simulink model "sfediticon"  (R2017b)
settings: Solver=FixedStepDiscrete  StartTime=0.0  StopTime=inf  RelTol=1e-3  EnableMultiTasking=on
CloseFcn:
  | sf_edit_icon('kill');
settings Model: FPTRunName=Active  ExtModeTrigMode=oneshot  ExtModeArmWhenConnect=off  ExtModeAutoUpdateStatusClock=off  Creator=The MathWorks, Inc.  LastModifiedBy=The MathWorks, Inc.
settings DataIOCC: SaveFormat=Array  SaveOutput=off  SaveTime=off
settings OptimizationCC: BooleanDataType=off  ExpressionDepthLimit=2147483647  InitFltsAndDblsToZero=on  EfficientMapNaN2IntZero=off  LifeSpan=inf
settings DebuggingCC: SaveWithParameterizedLinksMsg=none  UnderspecifiedInitializationDetection=Classic  MergeDetectMultiDrivingBlocksExec=none  SignalResolutionControl=TryResolveAllWithWarning  MultiTaskDSMMsg=warning  MultiTaskCondExecSysMsg=none  FcnCallInpInsideContextMsg=warning  StateNameClashWarn=warning  StrictBusMsg=None  SFUnexpectedBacktrackingDiag=warning  SFNoUnconditionalDefaultTransitionDiag=warning  SFExecutionAtInitializationDiag=none
settings HardwareCC: ProdBitPerPointer=32  ProdBitPerSizeT=32  ProdBitPerPtrDiffT=32  ProdLargestAtomicFloat=None  ProdIntDivRoundTo=Undefined  ProdEndianess=Unspecified  ProdWordSize=32  ProdHWDeviceType=32-bit Generic  TargetUnknown=on
settings ModelReferenceCC: PropagateSignalLabelsOutOfModel=off
settings SFSimCC: SimCustomHeaderCode=#define IS_MEX_TARGET 0  SimParseCustomCode=off
settings CodeAppCC: StateflowObjectComments=on
settings GRTTargetCC: TargetFcnLib=ansi_tfl_tmw.mat  TargetLangStandard=C89/C90 (ANSI)  GeneratePreprocessorConditionals=Disable all  CombineOutputUpdateFcns=off  GRTInterface=on
settings ConfigComp: CovMetricSettings=dcmtr  CovHtmlReporting=on  CovSaveCumulativeToWorkspaceVar=on  CovSaveSingleToWorkspaceVar=on  CovExternalEMLEnable=off  CovSFcnEnable=off

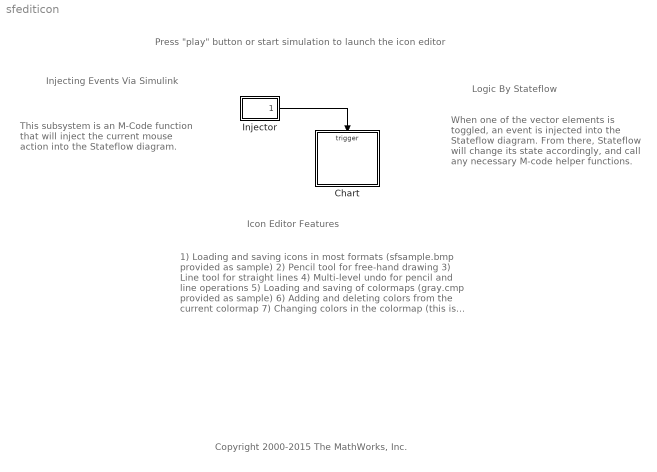
== system sfediticon ==
  note: This subsystem is an M-Code
      | function that will inject the
      | current mouse action into the
      | Stateflow diagram.
  note: Injecting Events
      | Via Simulink
  note: When one of the vector elements
      | is toggled, an event is injected
      | into the Stateflow diagram.
      | From there, Stateflow will
      | change its state accordingly,
      | and call any necessary M-code
      | helper functions.
  note: Logic By Stateflow
  note: 1) Loading and saving icons in most formats
      |      (sfsample.bmp provided as sample)
      | 2) Pencil tool for free-hand drawing
      | 3) Line tool for straight lines
      | 4) Multi-level undo for pencil and line operations
      | 5) Loading and saving of colormaps
      |      (gray.cmp provided as sample)
      | 6) Adding and deleting colors from the current
      |      colormap
      | 7) Changing colors in the colormap
      |     (this is immediately reflected in the icon)
  note: Icon Editor Features
  note: Press "play" button or start simulation to launch the icon editor
  note: Copyright 2000-2015 The MathWorks, Inc.
  Chart : Stateflow chart  TreatAsAtomicUnit=on
  Injector : Subsystem
  wires:
  Injector/1(Event) -> Chart/Trigger

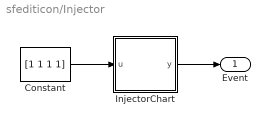
== system sfediticon/Injector ==
  Constant : Constant  Value=[1 1 1 1]
  InjectorChart : Stateflow chart  TreatAsAtomicUnit=on
  Event : Outport
  wires:
  InjectorChart/1(y) -> Event/1
  Constant/1 -> InjectorChart/1(u)

== stateflow chart sfediticon/Chart ==
  settings: executeAtInitialization=1
  state Main [parallel]
    settings: executionOrder=1
    state LineDraw
      en: ml.sf_edit_icon('anchor_line');
      du: ml.sf_edit_icon('render_line');
      ex:  ml.sf_edit_icon('commit');
    state Idle
    state PencilDraw
      en: ml.sf_edit_icon('draw_point');
      du: ml.sf_edit_icon('draw_point');
      ex:  ml.sf_edit_icon('commit');
    state FGColorSelect
      en: ml.sf_edit_icon('cache_color');
      ex: ml.sf_edit_icon('fgcolor');
    (default) -> Idle : {ml.sf_edit_icon('create');}
    (junction 125) -> LineDraw [order 1] : [pressedIcon == LINE_ICON]
    (junction 125) -> PencilDraw [order 2] : [pressedIcon == PENCIL_ICON]
    Idle -> (junction 125) [order 1] : NBD[in(ToolBar.Locked)&&...
        |          in(Focus.Canvas)]
    Main -> Idle : BU
    Idle -> FGColorSelect [order 2] : NBD[in(Focus.Palette.Swatch)]
    Idle -> (junction 132) [order 3] : ABD[in(Focus.Palette.Swatch)]
        | {ml.sf_edit_icon('show_color_menu');}
  state Focus [parallel]
    settings: executionOrder=2
    state Canvas
    state Icon
    state None
    state Palette
      state None
      state Swatch
      (junction 110) -> Focus.Palette.None [order 2]
      (junction 110) -> Swatch [order 1] : [ml.sf_edit_icon...
          | ('over_color_swatch')]
    state set_focusedIcon() [function]
      (default) -> (junction 113)
      (junction 113) -> (junction 114) [order 1] : [ml.sf_edit_icon('over_open_tool')] ...
          | {focusedIcon = OPEN_ICON;}
      (junction 113) -> (junction 115) [order 2]
      (junction 115) -> (junction 116) [order 1] : [ml.sf_edit_icon('over_saveas_tool')]...
          | {focusedIcon = SAVE_ICON;}
      (junction 115) -> (junction 117) [order 2]
      (junction 117) -> (junction 118) [order 1] : [ml.sf_edit_icon('over_openmap_tool')]...
          |  {focusedIcon = OPEN_MAP_ICON;}
      (junction 117) -> (junction 120) [order 2]
      (junction 120) -> (junction 119) [order 1] : [ml.sf_edit_icon('over_savemap_tool')] ...
          | {focusedIcon = SAVE_MAP_ICON;}
      (junction 120) -> (junction 121) [order 2]
      (junction 121) -> (junction 122) [order 1] : [ml.sf_edit_icon('over_undo_tool')]...
          |  {focusedIcon = UNDO_ICON;}
      (junction 121) -> (junction 128) [order 2]
      (junction 128) -> (junction 129) [order 1] : [ml.sf_edit_icon('over_line_tool')]...
          |  {focusedIcon = LINE_ICON;}
      (junction 128) -> (junction 130) [order 2]
      (junction 130) -> (junction 131) [order 1] : [ml.sf_edit_icon('over_pencil_tool')]...
          |  {focusedIcon = PENCIL_ICON;}
      (junction 130) -> (junction 112) [order 2] : {focusedIcon = 0;}
    state Toolbar
      en: set_focusedIcon();
      du: set_focusedIcon();
      ex: focusedIcon = 0;
    (default) -> Focus.None
    (junction 106) -> Canvas [order 1] : [ml.sf_edit_icon('over_canvas')]
    (junction 106) -> Icon [order 4] : [ml.sf_edit_icon('over_icon')]
    (junction 106) -> Focus.None [order 5]
    (junction 106) -> (junction 110) [order 2] : [ml.sf_edit_icon('over_palette')]
    Focus -> (junction 106) : BM
    (junction 106) -> (junction 133) [order 3] : [ml.sf_edit_icon('over_toolbar')]
    (junction 133) -> (junction 124) [order 1] : [in(Toolbar)]
    (junction 133) -> Toolbar [order 2]
  note: Note:
      | Make sure "Focus" comes before "Tool".
      | The Tool state depends on up-to-date
      | information about the Focus.
  state ToolBar [parallel]
    settings: executionOrder=3
    state press(icon,sp) [function]
      (default) -> (junction 126)
      (junction 126) -> (junction 104) [order 1] : [icon == OPEN_ICON] {ml.sf_edit_icon('press', sp, 'open');}
      (junction 126) -> (junction 105) [order 2]
      (junction 105) -> (junction 101) [order 1] : [icon == SAVE_ICON] {ml.sf_edit_icon('press', sp, 'save_as');}
      (junction 105) -> (junction 100) [order 2]
      (junction 100) -> (junction 102) [order 1] : [icon == OPEN_MAP_ICON] {ml.sf_edit_icon('press',sp,'open_map');}
      (junction 100) -> (junction 103) [order 2]
      (junction 103) -> (junction 109) [order 1] : [icon == SAVE_MAP_ICON] {ml.sf_edit_icon('press', sp, 'save_map');}
      (junction 103) -> (junction 111) [order 2]
      (junction 111) -> (junction 108) [order 1] : [icon == UNDO_ICON] {ml.sf_edit_icon('press',sp,'undo');}
      (junction 111) -> (junction 107) [order 2]
      (junction 107) -> (junction 123) [order 1] : [icon == LINE_ICON] {ml.sf_edit_icon('press',sp,'line');}
      (junction 107) -> (junction 90) [order 2]
      (junction 90) -> (junction 134) : [icon == PENCIL_ICON] {ml.sf_edit_icon('press',sp,'pencil');}
    state None
      pressedIcon = 0;
      ml.sf_edit_icon('status', 'Select a tool');
      ml.sf_edit_icon('normal_cursor');
    state Released
    state Pressed
      en:
      pressedIcon = focusedIcon;
      press(pressedIcon,1);
      ex: press(pressedIcon,0);
    state icon_operation(icon) [function]
      (default) -> (junction 91)
      (junction 91) -> (junction 93) [order 1] : [icon == OPEN_ICON] {ml.sf_edit_icon('open');}
      (junction 91) -> (junction 92) [order 2]
      (junction 92) -> (junction 94) [order 1] : [icon == SAVE_ICON] {ml.sf_edit_icon('save_as');}
      (junction 92) -> (junction 95) [order 2]
      (junction 95) -> (junction 96) [order 1] : [icon == OPEN_MAP_ICON] {ml.sf_edit_icon('open_map');}
      (junction 95) -> (junction 98) [order 2]
      (junction 98) -> (junction 97) [order 1] : [icon == SAVE_MAP_ICON] {ml.sf_edit_icon('save_map');}
      (junction 98) -> (junction 99) [order 2]
      (junction 99) -> (junction 135) : [icon == UNDO_ICON] {ml.sf_edit_icon('undo');}
    state Locked
      en:
      ml.sf_edit_icon...
      ('status', 'Tool locked');
    Released -> ToolBar.None [order 2] : BU
    (default) -> ToolBar.None
    (junction 127) -> ToolBar.None [order 3] : {icon_operation(pressedIcon);}
    ToolBar.None -> Pressed : NBD [in(Focus.Toolbar)]
    Pressed -> Released [order 1] : BM [pressedIcon != focusedIcon]
    Released -> Pressed [order 1] : BM [pressedIcon == focusedIcon]
    Pressed -> (junction 127) [order 2] : BU
    (junction 127) -> Locked [order 1] : [(pressedIcon == LINE_ICON)]...
        | {ml.sf_edit_icon('line_cursor');}
    (junction 127) -> Locked [order 2] : [(pressedIcon == PENCIL_ICON)]...
        | {ml.sf_edit_icon('pencil_cursor');}
    Locked -> Pressed : NBD[in(Focus.Toolbar)]
  data: icon function_input double; sp function_input double; icon function_input double; LINE_ICON constant int32 =1; OPEN_ICON constant int32 =2; OPEN_MAP_ICON constant int32 =3; PENCIL_ICON constant int32 =4; SAVE_MAP_ICON constant int32 =5; UNDO_ICON constant int32 =6; pressedIcon local int32; focusedIcon local int32; SAVE_ICON constant int32 =7
  events: BM input EITHER_EDGE_EVENT; NBD input EITHER_EDGE_EVENT; BU input EITHER_EDGE_EVENT; ABD input EITHER_EDGE_EVENT

== stateflow chart sfediticon/Injector/InjectorChart ==
  (default) -> (junction 2) : {y = ml.sf_inject_event(u);}
  data: u input; y output
